simulink model "ANS_GFM_short_term"  (R2021b)
settings: Solver=FixedStepAuto  StartTime=0.0  StopTime=5  FixedStep=Ts  MaxStep=1e-5  RelTol=1e-3
values from neighbouring files (symbols this model uses):
  angle_load = angle(LF.bus(ind_l).Vbus)*180/pi    [init_ANS_GFM_long_term.m]    (also in init_ANS_GFM_short_term.m)
  angleV_LF = Vangle_init/180*pi    [init_ANS_GFM_long_term.m]    (also in init_ANS_GFM_short_term.m)
  awu = 1    [init_ANS_GFM_long_term.m]    (also in init_ANS_GFM_short_term.m)
  C_dc = 1/(Xcdc_pu_or*Zbase_dc_new*100*pi)    [init_ANS_GFM_long_term.m]    (also in init_ANS_GFM_short_term.m)
  C_f = 1/(Xcf_pu_or*Zbase_new*100*pi)    (= 0.013712)    [init_ANS_GFM_long_term.m]    (also in init_ANS_GFM_short_term.m = 0.0141333333333)
  control = 3    [init_ANS_GFM_long_term.m]    (also in init_ANS_GFM_short_term.m = 1)
  D_p = (1/(m_p*w_b))    (= 5209935.26289)    [init_ANS_GFM_long_term.m]    (also in init_ANS_GFM_short_term.m = 5370022.73304)
  Egrid_tmp = 1.054080675694902*400e3    (= 421632.270278)    [init_ANS_GFM_long_term.m]    (also in init_ANS_GFM_short_term.m)
  epsi = 1e-4    (= 0.0001)    [init_ANS_GFM_long_term.m]    (also in init_ANS_GFM_short_term.m)
  eta = m_p*V_m^2    [init_ANS_GFM_long_term.m]    (also in init_ANS_GFM_short_term.m)
  gamma = 2.3    [init_ANS_GFM_long_term.m]    (also in init_ANS_GFM_short_term.m)
  I0_init = [I0_init_a, I0_init_b, I0_init_c]    [init_ANS_GFM_long_term.m]    (also in init_ANS_GFM_short_term.m)
  I_bc = S_bc / (V_bc*sqrt(3))    [init_ANS_GFM_long_term.m]    (also in init_ANS_GFM_short_term.m)
  I_d_int_init = (U_d_int + I_q_int*L_f*w_b - V_d_int - I_d_int*R_f*0)    [init_ANS_GFM_long_term.m]    (also in init_ANS_GFM_short_term.m)
  I_init = [I_init_a, I_init_b, I_init_c]    [init_ANS_GFM_long_term.m]    (also in init_ANS_GFM_short_term.m)
  i_ll = -1.15*(S_bc/Vdc_n)-i_loss_dc    [init_ANS_GFM_long_term.m]    (also in init_ANS_GFM_short_term.m)
  I_max_sat_pu = 1.0 * I_bc *sqrt(2)    [init_ANS_GFM_long_term.m]    (also in init_ANS_GFM_short_term.m)
  I_q_int_init = (U_q_int - I_d_int*L_f*w_b - V_q_int - I_q_int*R_f*0)    [init_ANS_GFM_long_term.m]    (also in init_ANS_GFM_short_term.m)
  i_ul = 1.15*(S_bc/Vdc_n)+i_loss_dc    [init_ANS_GFM_long_term.m]    (also in init_ANS_GFM_short_term.m)
  idppu = 0.95    [init_ANS_GFM_long_term.m]    (also in init_ANS_GFM_short_term.m = 0.92)
  init_dP = -inv(A_pm)*B_pm*dP    [init_ANS_GFM_long_term.m]    (also in init_ANS_GFM_short_term.m)
  init_pm = -inv(A_pm)*B_pm*P_aft    [init_ANS_GFM_long_term.m]    (also in init_ANS_GFM_short_term.m)
  init_tau = -inv(A_tau)*B_tau*idc    [init_ANS_GFM_long_term.m]    (also in init_ANS_GFM_short_term.m)
  J = D_p*tau_f    (= 104198.705258)    [init_ANS_GFM_long_term.m]    (also in init_ANS_GFM_short_term.m = 107400.454661)
  k_dc = eta_1/(Vdc_n*m_p)    [init_ANS_GFM_long_term.m]    (also in init_ANS_GFM_short_term.m)
  K_p = (1/Vdc_n)    [init_ANS_GFM_long_term.m]    (also in init_ANS_GFM_short_term.m)
  K_r = 1/R_dc    [init_ANS_GFM_long_term.m]    (also in init_ANS_GFM_short_term.m)
  Kff_i = 1    [init_ANS_GFM_long_term.m]    (also in init_ANS_GFM_short_term.m)
  Kff_v = 1    [init_ANS_GFM_long_term.m]    (also in init_ANS_GFM_short_term.m)
  Ki_i = (1/n)*1.19    (= 0.0520711785298)    [init_ANS_GFM_long_term.m]    (also in init_ANS_GFM_short_term.m = 0.0505188679245)
  Ki_pll = 4255.3    [init_ANS_GFM_long_term.m]    (also in init_ANS_GFM_short_term.m)
  Ki_v = (n)*1.161022    (= 26.5332227733)    [init_ANS_GFM_long_term.m]    (also in init_ANS_GFM_short_term.m = 27.3485182222)
  ki_v_ac = 2*0.25    (= 0.5)    [init_ANS_GFM_long_term.m]    (also in init_ANS_GFM_short_term.m)
  Kp_i = 0.738891/n    (= 0.032331869895)    [init_ANS_GFM_long_term.m]    (also in init_ANS_GFM_short_term.m = 0.0313680141509)
  Kp_pll = 92    [init_ANS_GFM_long_term.m]    (also in init_ANS_GFM_short_term.m)
  Kp_v = 0.52*n    (= 11.8837333333)    [init_ANS_GFM_long_term.m]    (also in init_ANS_GFM_short_term.m = 12.2488888889)
  kp_v_ac = 0.001    [init_ANS_GFM_long_term.m]    (also in init_ANS_GFM_short_term.m)
  Kpl = 5.0    (= 5)    [init_ANS_GFM_long_term.m]    (also in init_ANS_GFM_short_term.m)
  L1 = cf/sqrt(1+RX^2)*(400e3)^2/Skss/(100*pi)    [init_ANS_GFM_long_term.m]    (also in init_ANS_GFM_short_term.m)
  L_f = Xlf_pu_or*Zbase_new/100/pi    (= 4.37572928821e-06)    [init_ANS_GFM_long_term.m]    (also in init_ANS_GFM_short_term.m = 4.24528301887e-06)
  Lf = 1e6/100/pi    (= 3183.09886184)    [init_ANS_GFM_long_term.m]    (also in init_ANS_GFM_short_term.m = 0.0636619772368)
  m_p = (2*pi*0.5)/(S_bc)    (= 6.10967066042e-10)    [init_ANS_GFM_long_term.m]    (also in init_ANS_GFM_short_term.m = 5.92753330866e-10)
  n = 1/Zb    (= 22.8533333333)    [init_ANS_GFM_long_term.m]    (also in init_ANS_GFM_short_term.m = 23.5555555556)
  P_LF_si = P_LF*S_b    [init_ANS_GFM_long_term.m]    (also in init_ANS_GFM_short_term.m)
  ps = 4440e6/S_bc    (= 0.863477246208)    [init_ANS_GFM_long_term.m]    (also in init_ANS_GFM_short_term.m = 0.837735849057)
  Q_LF_si = Q_LF*S_b    [init_ANS_GFM_long_term.m]    (also in init_ANS_GFM_short_term.m)
  qs = Q_LF*S_b/S_bc    [init_ANS_GFM_long_term.m]    (also in init_ANS_GFM_short_term.m)
  R1 = RX*cf/sqrt(1+RX^2)*(400e3)^2/Skss    [init_ANS_GFM_long_term.m]    (also in init_ANS_GFM_short_term.m)
  R_dc = Rdc_pu_or*Zbase_dc_new    [init_ANS_GFM_long_term.m]    (also in init_ANS_GFM_short_term.m)
  R_f = Rf_pu_or*Zbase_new    (= 2.18786464411e-05)    [init_ANS_GFM_long_term.m]    (also in init_ANS_GFM_short_term.m = 2.12264150943e-05)
  Rf = 1e6    (= 1000000)    [init_ANS_GFM_long_term.m]    (also in init_ANS_GFM_short_term.m = 20)
  S_bc = 5142e6    (= 5142000000)    [init_ANS_GFM_long_term.m]    (also in init_ANS_GFM_short_term.m = 5300000000)
  sat_select = 3    [init_ANS_GFM_long_term.m]    (also in init_ANS_GFM_short_term.m)
  SECM = 3    [init_ANS_GFM_long_term.m]    (also in init_ANS_GFM_short_term.m = 1)
  share_i_load = 1.0    (= 1)    [init_ANS_GFM_long_term.m]    (also in init_ANS_GFM_short_term.m)
  T_en = -0.5    [init_ANS_GFM_long_term.m]    (also in init_ANS_GFM_short_term.m)
  T_off = T_on + 0.1    (= 0.2)    [init_ANS_GFM_long_term.m]    (also in init_ANS_GFM_short_term.m)
  T_on = 0.1    [init_ANS_GFM_long_term.m]    (also in init_ANS_GFM_short_term.m)
  Ts = 2e-6    (= 2e-06)    [init_ANS_GFM_long_term.m]    (also in init_ANS_GFM_short_term.m = 1e-06)
  U_init = [Umag_init_a, Umag_init_b, Umag_init_c]    [init_ANS_GFM_long_term.m]    (also in init_ANS_GFM_short_term.m)
  Uangle_init = angle(V_LF_VSC)*180/pi    [init_ANS_GFM_long_term.m]    (also in init_ANS_GFM_short_term.m)
  Umag_init = abs(V_LF_VSC)*V_bc*sqrt(2/3)    [init_ANS_GFM_long_term.m]    (also in init_ANS_GFM_short_term.m)
  V1_rms = 15e3    (= 15000)    [init_ANS_GFM_long_term.m]    (also in init_ANS_GFM_short_term.m)
  V_d_int = abs(V_LF)*V_bc*sqrt(2/3)    [init_ANS_GFM_long_term.m]    (also in init_ANS_GFM_short_term.m)
  V_d_int_init = (I_d_int + V_q_int*C_f*w_b - I0_d_int)    [init_ANS_GFM_long_term.m]    (also in init_ANS_GFM_short_term.m)
  V_init = [V_init_a, V_init_b, V_init_c]    [init_ANS_GFM_long_term.m]    (also in init_ANS_GFM_short_term.m)
  V_m = sqrt(2/3)*V_bc    [init_ANS_GFM_long_term.m]    (also in init_ANS_GFM_short_term.m)
  V_q_int_init = (I_q_int - V_d_int*C_f*w_b - I0_q_int)    [init_ANS_GFM_long_term.m]    (also in init_ANS_GFM_short_term.m)
  Vdc_n = 3*V_m    [init_ANS_GFM_long_term.m]    (also in init_ANS_GFM_short_term.m)
  Vref = V_LF_mag*V_m    [init_ANS_GFM_long_term.m]    (also in init_ANS_GFM_short_term.m)
  w_b = 2*pi*f_b    (= 314.159265359)    [init_ANS_GFM_long_term.m]    (also in init_ANS_GFM_short_term.m)
  w_f = 2*pi*5    (= 31.4159265359)    [init_ANS_GFM_long_term.m]    (also in init_ANS_GFM_short_term.m)
  Zbase_new = V1_rms^2/S_bc    (= 0.0437572928821)    [init_ANS_GFM_long_term.m]    (also in init_ANS_GFM_short_term.m = 0.0424528301887)
undefined symbols (not defined in the file or in its folder): A_pm, A_tau, B_pm, B_tau, C_pm, C_tau, D_pm, D_tau, find_system, idq0_init, Pm, sm_init, v_d, v_q, Ve
libraries: spsBreakerLib x270, spsGroundLib x21, spsThreePhaseSeriesRLCBranchLib x12, spsabctodq0Lib x11, simulink x9, spsEdgeDetectorLib x8, spsThreePhaseVIMeasurementLib x7, spsLoadFlowBusLib x7, spsSeriesRLCBranchLib x6, spsControlledVoltageSourceLib x6, spsCurrentMeasurementLib x6, spsVoltageMeasurementLib x6
(part 6 of 7)

== system ANS_GFM_short_term/OLTC for load flow/OLTCC1 ==
  note: R2
  note: R1
  note: Transfer Switch
  Demux : Demux  Outputs=21
      settings: DisplayOption=none
  Display : Display
  Display1 : Display
  "Sw0 " : spsBreakerLib/Breaker  InitialState=InitialStates(1)  SwitchingTimes="[ 1/60  5/60 ]"  External=on  BreakerResistance=1e-6  SnubberResistance=1e8  SnubberCapacitance=inf  Measurements=None  MoreParameters=off  NoBreakLoop=off
      settings: SourceProductBaseCode=PS
  "Sw1 " : spsBreakerLib/Breaker  InitialState=InitialStates(2)  SwitchingTimes="[ 1/60  5/60 ]"  External=on  BreakerResistance=1e-4  SnubberResistance=1e6  SnubberCapacitance=inf  Measurements=None  MoreParameters=off  NoBreakLoop=off
      settings: SourceProductBaseCode=PS
  Sw10 : spsBreakerLib/Breaker  InitialState=InitialStates(11)  SwitchingTimes="[ 1/60  5/60 ]"  External=on  BreakerResistance=1e-6  SnubberResistance=1e8  SnubberCapacitance=inf  Measurements=None  MoreParameters=off  NoBreakLoop=off
      settings: SourceProductBaseCode=PS
  Sw11 : spsBreakerLib/Breaker  InitialState=InitialStates(12)  SwitchingTimes="[ 1/60  5/60 ]"  External=on  BreakerResistance=1e-6  SnubberResistance=1e8  SnubberCapacitance=inf  Measurements=None  MoreParameters=off  NoBreakLoop=off
      settings: SourceProductBaseCode=PS
  Sw12 : spsBreakerLib/Breaker  InitialState=InitialStates(13)  SwitchingTimes="[ 1/60  5/60 ]"  External=on  BreakerResistance=1e-6  SnubberResistance=1e8  SnubberCapacitance=inf  Measurements=None  MoreParameters=off  NoBreakLoop=off
      settings: SourceProductBaseCode=PS
  Sw13 : spsBreakerLib/Breaker  InitialState=InitialStates(14)  SwitchingTimes="[ 1/60  5/60 ]"  External=on  BreakerResistance=1e-4  SnubberResistance=1e6  SnubberCapacitance=inf  Measurements=None  MoreParameters=off  NoBreakLoop=off
      settings: SourceProductBaseCode=PS
  Sw14 : spsBreakerLib/Breaker  InitialState=InitialStates(15)  SwitchingTimes="[ 1/60  5/60 ]"  External=on  BreakerResistance=1e-4  SnubberResistance=1e6  SnubberCapacitance=inf  Measurements=None  MoreParameters=off  NoBreakLoop=off
      settings: SourceProductBaseCode=PS
  Sw15 : spsBreakerLib/Breaker  InitialState=InitialStates(16)  SwitchingTimes="[ 1/60  5/60 ]"  External=on  BreakerResistance=1e-4  SnubberResistance=1e6  SnubberCapacitance=inf  Measurements=None  MoreParameters=off  NoBreakLoop=off
      settings: SourceProductBaseCode=PS
  Sw16 : spsBreakerLib/Breaker  InitialState=InitialStates(17)  SwitchingTimes="[ 1/60  5/60 ]"  External=on  BreakerResistance=1e-4  SnubberResistance=1e6  SnubberCapacitance=inf  Measurements=None  MoreParameters=off  NoBreakLoop=off
      settings: SourceProductBaseCode=PS
  Sw17 : spsBreakerLib/Breaker  InitialState=InitialStates(18)  SwitchingTimes="[ 1/60  5/60 ]"  External=on  BreakerResistance=1e-4  SnubberResistance=1e6  SnubberCapacitance=inf  Measurements=None  MoreParameters=off  NoBreakLoop=off
      settings: SourceProductBaseCode=PS
  Sw18 : spsBreakerLib/Breaker  InitialState=InitialStates(19)  SwitchingTimes="[ 1/60  5/60 ]"  External=on  BreakerResistance=1e-4  SnubberResistance=1e6  SnubberCapacitance=inf  Measurements=None  MoreParameters=off  NoBreakLoop=off
      settings: SourceProductBaseCode=PS
  Sw19 : spsBreakerLib/Breaker  InitialState=InitialStates(20)  SwitchingTimes="[ 1/60  5/60 ]"  External=on  BreakerResistance=1e-4  SnubberResistance=1e6  SnubberCapacitance=inf  Measurements=None  MoreParameters=off  NoBreakLoop=off
      settings: SourceProductBaseCode=PS
  "Sw2 " : spsBreakerLib/Breaker  InitialState=InitialStates(3)  SwitchingTimes="[ 1/60  5/60 ]"  External=on  BreakerResistance=1e-4  SnubberResistance=1e6  SnubberCapacitance=inf  Measurements=None  MoreParameters=off  NoBreakLoop=off
      settings: SourceProductBaseCode=PS
  Sw20 : spsBreakerLib/Breaker  InitialState=InitialStates(21)  SwitchingTimes="[ 1/60  5/60 ]"  External=on  BreakerResistance=1e-4  SnubberResistance=1e6  SnubberCapacitance=inf  Measurements=None  MoreParameters=off  NoBreakLoop=off
      settings: SourceProductBaseCode=PS
  "Sw3 " : spsBreakerLib/Breaker  InitialState=InitialStates(4)  SwitchingTimes="[ 1/60  5/60 ]"  External=on  BreakerResistance=1e-4  SnubberResistance=1e6  SnubberCapacitance=inf  Measurements=None  MoreParameters=off  NoBreakLoop=off
      settings: SourceProductBaseCode=PS
  "Sw4 " : spsBreakerLib/Breaker  InitialState=InitialStates(5)  SwitchingTimes="[ 1/60  5/60 ]"  External=on  BreakerResistance=1e-4  SnubberResistance=1e6  SnubberCapacitance=inf  Measurements=None  MoreParameters=off  NoBreakLoop=off
      settings: SourceProductBaseCode=PS
  "Sw5 " : spsBreakerLib/Breaker  InitialState=InitialStates(6)  SwitchingTimes="[ 1/60  5/60 ]"  External=on  BreakerResistance=1e-4  SnubberResistance=1e6  SnubberCapacitance=inf  Measurements=None  MoreParameters=off  NoBreakLoop=off
      settings: SourceProductBaseCode=PS
  "Sw6 " : spsBreakerLib/Breaker  InitialState=InitialStates(7)  SwitchingTimes="[ 1/60  5/60 ]"  External=on  BreakerResistance=1e-6  SnubberResistance=1e8  SnubberCapacitance=inf  Measurements=None  MoreParameters=off  NoBreakLoop=off
      settings: SourceProductBaseCode=PS
  "Sw7 " : spsBreakerLib/Breaker  InitialState=InitialStates(8)  SwitchingTimes="[ 1/60  5/60 ]"  External=on  BreakerResistance=1e-6  SnubberResistance=1e68  SnubberCapacitance=inf  Measurements=None  MoreParameters=off  NoBreakLoop=off
      settings: SourceProductBaseCode=PS
  "Sw8 " : spsBreakerLib/Breaker  InitialState=InitialStates(9)  SwitchingTimes="[ 1/60  5/60 ]"  External=on  BreakerResistance=1e-6  SnubberResistance=1e8  SnubberCapacitance=inf  Measurements=None  MoreParameters=off  NoBreakLoop=off
      settings: SourceProductBaseCode=PS
  Sw9 : spsBreakerLib/Breaker  InitialState=InitialStates(10)  SwitchingTimes="[ 1/60  5/60 ]"  External=on  BreakerResistance=1e-6  SnubberResistance=1e8  SnubberCapacitance=inf  Measurements=None  MoreParameters=off  NoBreakLoop=off
      settings: SourceProductBaseCode=PS
  SwR1 : spsBreakerLib/Breaker  InitialState=1  SwitchingTimes="[ 1/60  5/60 ]"  External=on  BreakerResistance=1e-6  SnubberResistance=Rtransfer  SnubberCapacitance=inf  Measurements=None  MoreParameters=off  NoBreakLoop=off
      settings: SourceProductBaseCode=PS
  SwR2 : spsBreakerLib/Breaker  InitialState=1  SwitchingTimes="[ 1/60  5/60 ]"  External=on  BreakerResistance=1e-6  SnubberResistance=Rtransfer  SnubberCapacitance=inf  Measurements=None  MoreParameters=off  NoBreakLoop=off
      settings: SourceProductBaseCode=PS
  Tapped Winding Inversion : Subsystem
  Tap20 : PMIOPort  Side=Right
  Tap19 : PMIOPort  Port=2  Side=Right
  Tap18 : PMIOPort  Port=3  Side=Right
  Tap17 : PMIOPort  Port=4  Side=Right
  Tap16 : PMIOPort  Port=5  Side=Right
  Tap15 : PMIOPort  Port=6  Side=Right
  Tap14 : PMIOPort  Port=7  Side=Right
  Tap13 : PMIOPort  Port=8  Side=Right
  Tap12 : PMIOPort  Port=9  Side=Right
  Tap11 : PMIOPort  Port=10  Side=Right
  Tap10 : PMIOPort  Port=11  Side=Right
  Tap9 : PMIOPort  Port=12  Side=Right
  Tap8 : PMIOPort  Port=13  Side=Right
  Tap7 : PMIOPort  Port=14  Side=Right
  Tap6 : PMIOPort  Port=15  Side=Right
  Tap5 : PMIOPort  Port=16  Side=Right
  Tap4 : PMIOPort  Port=17  Side=Right
  Tap3 : PMIOPort  Port=18  Side=Right
  Tap2 : PMIOPort  Port=19  Side=Right
  Tap1 : PMIOPort  Port=20  Side=Right
  Tap0 : PMIOPort  Port=21  Side=Right
  W2+ : PMIOPort  Port=22  Side=Right
  Out : PMIOPort  Port=23  Side=Left
  wires:
  Demux/9 -> "Sw8 "/1
  Demux/8 -> "Sw7 "/1
  Demux/7 -> Display/1, "Sw6 "/1
  Demux/6 -> "Sw5 "/1
  Demux/5 -> "Sw4 "/1
  Demux/4 -> "Sw3 "/1
  Demux/3 -> "Sw2 "/1
  Demux/2 -> "Sw1 "/1
  Demux/1 -> "Sw0 "/1
  [SwInversion] -> Tapped Winding Inversion/1(Inv)
  [SwTransfer] -> SwR2/1, SwR1/1
  [SwSelect] -> Demux/1, Display1/1
  Demux/10 -> Sw9/1
  Demux/11 -> Sw10/1
  Demux/12 -> Sw11/1
  Demux/13 -> Sw12/1
  Demux/14 -> Sw13/1
  Demux/15 -> Sw14/1
  Demux/16 -> Sw15/1
  Demux/17 -> Sw16/1
  Demux/18 -> Sw17/1
  Demux/19 -> Sw18/1
  Demux/20 -> Sw19/1
  Demux/21 -> Sw20/1
  connections:
  "Sw0 "/LConn1 -- Tap0/RConn1 -- Tapped Winding Inversion/LConn2
  Tap1/RConn1 -- "Sw1 "/LConn1
  Tap2/RConn1 -- "Sw2 "/LConn1
  Tap6/RConn1 -- "Sw6 "/LConn1
  Tap4/RConn1 -- "Sw4 "/LConn1
  Tap5/RConn1 -- "Sw5 "/LConn1
  SwR1/RConn1 -- Tapped Winding Inversion/LConn1 -- SwR2/RConn1
  SwR2/LConn1 -- Sw19/RConn1 -- Sw17/RConn1 -- Sw15/RConn1 -- Sw13/RConn1 -- Sw11/RConn1 -- Sw9/RConn1 -- "Sw7 "/RConn1 -- "Sw5 "/RConn1 -- "Sw3 "/RConn1 -- "Sw1 "/RConn1
  Tapped Winding Inversion/RConn1 -- Out/RConn1
  W2+/RConn1 -- Tapped Winding Inversion/RConn2
  "Sw6 "/RConn1 -- "Sw4 "/RConn1 -- "Sw2 "/RConn1 -- "Sw0 "/RConn1 -- Sw20/RConn1 -- Sw18/RConn1 -- Sw16/RConn1 -- Sw14/RConn1 -- Sw12/RConn1 -- Sw10/RConn1 -- "Sw8 "/RConn1 -- SwR1/LConn1
  Tap3/RConn1 -- "Sw3 "/LConn1
  Tap8/RConn1 -- "Sw8 "/LConn1
  Tap7/RConn1 -- "Sw7 "/LConn1
  Tap9/RConn1 -- Sw9/LConn1
  Tap10/RConn1 -- Sw10/LConn1
  Tap11/RConn1 -- Sw11/LConn1
  Tap13/RConn1 -- Sw13/LConn1
  Tap12/RConn1 -- Sw12/LConn1
  Tap14/RConn1 -- Sw14/LConn1
  Tap15/RConn1 -- Sw15/LConn1
  Tap16/RConn1 -- Sw16/LConn1
  Tap17/RConn1 -- Sw17/LConn1
  Tap18/RConn1 -- Sw18/LConn1
  Tap19/RConn1 -- Sw19/LConn1
  Tap20/RConn1 -- Sw20/LConn1

== system ANS_GFM_short_term/OLTC for load flow/Subsystem ==
  note: A) Open the Three-Phase OLTC Transformer  mask (use Edit/Edit mask)
      |      In Initialization section, modify 1st line as below:
      |                   NumberOfTaps=10;
      |
      | B) Open the TransformerA block dialog box inside the Three-Phase OLTC Transformer (use Edit/Look under mask)
      |      and change the 'Number of Taps' parameter  from 7 to 9 (adding two intermediate taps on upper left winding (winding 1)).
      |
      | C) Open the  OLTCA block inside the Three-Phase OLTC Transformer (use Edit/Look under mask) and make the following changes:
      |       1) Open the dialog box of the Demux block and change the parameter  'Number of outputs' from 9 to 11.
      |       2) Add 2 switches labeled Sw9 and Sw10 (duplicate Sw8 block); Position these two blocks on top of Sw8 block.
      |       3) Open the dialog box of Sw9 and Sw10 blocks and change the  parameter "Initial state" as follows:
      |              Sw9 --> InitialState(10)
      |              Sw10-->InitialState(11)
      |      4) Add two connection ports labeled  respectively Tap9 and Tap10 (duplicate Tap8 block). Position these two blocks on top of Tap8 block.
      |      5) Renumber ALL connection ports as follows:
      |         Open dialog box of each connection port and change  'Port number' and  'Port location' parameters as in the table below.
      |         (all port locations should be set to  'right' except for 'Out' port which must be 'left')
      |         Start the renumbering with the top port  labeled Tap10.
      |
      |            Port           Port          Port
      |            label       number   location
      |           ---------    -----------    -----------
      |            Tap10       1               right
      |            Tap9         2               right
      |            .....            ......              .......
      |            Tap 1       11               right
      |            Tap 0       12               right
      |            W2+         13               right
      |            Out           14               left
      |
      |     6) Connect terminal 1 of Sw9 and Sw10 respectively to ports labeled Tap10 (port #1)  and Tap9  (port #2)
      |     7) Connect terminal 2 of Sw9 and Sw10 respectively to nodes labeled R2 and R1
      |     8) Close the OLTCA block.
      |
      | D)  Connect the Tap10, Tap9 ...Tap0 connectors of OLTCA respectively to  1+, 1.1,   ... 1 connectors of tapped winding of TransformerA.
      |
      | E)  Cut  the OLTCB and OLTCC blocks and replace them with a duplicate of OLTCA block.  Rename these two blocks OLTCB and OLTCC.
      |
      | F)  Cut  the TransformerB and TransformerC blocks and replace them with a duplicate of TransformerA block. Rename these two blocks TransformerB and TransformerC.
      |
      | G) Make connections between OLTC to Transformer for  phases B and C as for phase A.
      |
      | H) Ckeck that the secondary windings of  the three transformers are connected in Delta (D1)
  note: The following procedure explains how to increase the number of taps from 8 (17 OLTC positions)  to 10  (21 OLTC positions)
      |    If you want to decrease the number of taps, follow the reverse procedure (Change 'add' to ' cut'  and skip step C3).

== system ANS_GFM_short_term/OLTC for load flow/Voltage regulator ==
  Vmes (pu) : Inport
  Ready : Inport  Port=2
  RegOn : Inport  Port=3
  Dead Zone : DeadZone  LowerValue=-DeadBand/2  UpperValue=+DeadBand/2  SaturateOnIntegerOverflow=on
  Logical Operator : Logic  AllPortsSameDT=off
  Logical Operator1 : Logic  AllPortsSameDT=off
  MyDelay1 : Subsystem
  MyDelay2 : Subsystem
  Relational Operator : RelationalOperator  Operator=>  RndMeth=Nearest
  Relational Operator1 : RelationalOperator  Operator=<  RndMeth=Nearest
  Sum : Sum  Inputs=|+-  SaturateOnIntegerOverflow=on
  Switch : Switch  Threshold=1.5  SaturateOnIntegerOverflow=on
  Transport Delay : TransportDelay  DelayTime=Ts  InitialOutput=1
  Vref : Constant  Value=Vref
  Vref1 : Constant  Value=0
  Vref2 : Constant  Value=0
  Vref3 : Constant  Value=0
  Up : Outport  VectorParamsAs1DForOutWhenUnconnected=off
  Down : Outport  Port=2  VectorParamsAs1DForOutWhenUnconnected=off
  wires:
  Vref2/1 -> Switch/3
  RegOn/1 -> Switch/2
  Switch/1 -> Dead Zone/1
  Sum/1 -> Switch/1
  Vref/1 -> Sum/1
  Vmes (pu)/1 -> Sum/2
  Dead Zone/1 -> Relational Operator1/1, Relational Operator/1
  Vref1/1 -> Relational Operator/2
  Relational Operator/1 -> Logical Operator/1
  Ready/1 -> Transport Delay/1
  Transport Delay/1 -> Logical Operator1/1, Logical Operator/2
  Relational Operator1/1 -> Logical Operator1/2
  Logical Operator1/1 -> MyDelay1/1(in)
  Vref3/1 -> Relational Operator1/2
  MyDelay2/1(out) -> Up/1
  MyDelay1/1(out) -> Down/1
  Logical Operator/1 -> MyDelay2/1(in)

== system ANS_GFM_short_term/Synchronous Generator(GENTPJ)/AVR+OEL+PSS ==
  ie : Inport
  ut : Inport  Port=2
  xspeed : Inport  Port=3
  Array logic : Subsystem
  Constant : Constant  Value=ifdlim
  Constant2 : Constant  Value=uref+ve0/G
  Constant3 : Constant  Value=PSS_act
  Constant4 : Constant  Value=0
  DT1-Glied : Subsystem  mask(State Space Model){A=-2/30, B=1, C=-1/3, D=5, x_init=-1*1/(-2/30)}
      mask prompts: x_init "Initialisierung (x_init)"
      mask help:
      | [A,B,C,D] = tf2ss([Kp],[Tw 1])
      |
      | Kp = 75
      | Tw = 15
      |
      | Initialisierung:
      |
      | x_init = -B*u/A
      |
      | --> u muss man zurückverfolgen, welchen Wert dieser hat
  Gain : Gain  Gain=-1
  Gain2 : Gain  Gain=10
  Integrator Limited : Integrator  InitialCondition=L1  LimitOutput=on  LowerSaturationLimit=L1
  Integrator Limited1 : Integrator  InitialCondition=ve0  LimitOutput=on  UpperSaturationLimit=L2  LowerSaturationLimit=0
  Lead-Lag : Subsystem  mask(State Space Model){A=-0.08, B=1, C=5.76, D=48, x_init=-1*ve0/G/(-0.08)}
      mask prompts: x_init "Initialisierung (x_init)"
      mask help:
      | [A,B,C,D] = tf2ss(120*[5 1],[12.5 1])
      |
      | Initialisierung:
      |
      | x_init = -B*u/A
      |
      | --> u muss man zurückverfolgen, welchen Wert dieser hat
  Lead_Lag1 : Subsystem  mask(State Space Model){A=-83-1/3, B=1, C=-1.4444e+03, D=18+1/3, x_init=-1*0/(-83-1/3)}
      mask prompts: x_init "Initialisierung (x_init)"
      mask help:
      | [A,B,C,D] = tf2ss([T1 1],[T2 1])
      |
      | T1 = 0.22
      | T2 = 0.012
      |
      | Initialisierung:
      |
      | x_init = -B*u/A
      |
      | --> u muss man zurückverfolgen, welchen Wert dieser hat
  Lead_Lag2 : Subsystem  mask(State Space Model){A=-83-1/3, B=1, C=-1.4444e+03, D=18+1/3, x_init=-1*0/(-83-1/3)}
      mask prompts: x_init "Initialisierung (x_init)"
      mask help:
      | [A,B,C,D] = tf2ss([T1 1],[T2 1])
      |
      | T1 = 0.22
      | T2 = 0.012
      |
      | Initialisierung:
      |
      | x_init = -B*u/A
      |
      | --> u muss man zurückverfolgen, welchen Wert dieser hat
  Min : MinMax  Inputs=2
  Mux : Mux  Commented=on  Inputs=2
  Saturation : Saturate  UpperLimit=C  LowerLimit=-C
  Sum : Sum  Inputs=|+-
  Sum1 : Sum  Inputs=+-+
  Sum2 : Sum  Inputs=|+-
  Switch1 : Switch  Criteria=u2 > Threshold
  Switch2 : Switch  Criteria=u2 > Threshold
  To Workspace : ToWorkspace  Commented=on  VariableName=oel  SaveFormat=Timeseries  SampleTime=-1
      settings: Decimation=100
  Transfer Fcn : TransferFcn  Commented=on  Numerator=[Ta 1]  Denominator=[Tb 1]
  Transfer Fcn1 : TransferFcn  Commented=on  Numerator=[Kp]  Denominator=[Tw 1]
  Transfer Fcn2 : TransferFcn  Commented=on  Numerator=[T1 1]  Denominator=[T2 1]
  Transfer Fcn3 : TransferFcn  Commented=on  Numerator=[T1 1]  Denominator=[T2 1]
  ve : Outport
  wires:
  Sum/1 -> Array logic/1(u), Gain/1
  Gain2/1 -> Integrator Limited1/1
  Sum1/1 -> Switch1/3, Min/2
  Integrator Limited1/1 -> ve/1, Sum2/2
  Switch2/1 -> Sum1/3
  Array logic/1(y) -> Mux/1, Integrator Limited/1
  Constant3/1 -> Switch2/2
  Saturation/1 -> Switch2/1
  Constant4/1 -> Switch2/3
  Min/1 -> Lead-Lag/1(u)
  Constant/1 -> Sum/2
  Integrator Limited/1 -> Mux/2, Switch1/2
  Gain/1 -> Switch1/1
  Switch1/1 -> Min/1
  ie/1 -> Sum/1
  Sum2/1 -> Gain2/1
  ut/1 -> Sum1/2
  Constant2/1 -> Sum1/1
  Lead-Lag/1(y) -> Sum2/1
  Transfer Fcn1/1 -> Transfer Fcn2/1
  Transfer Fcn2/1 -> Transfer Fcn3/1
  xspeed/1 -> DT1-Glied/1(u)
  DT1-Glied/1(y) -> Lead_Lag1/1(u)
  Lead_Lag1/1(y) -> Lead_Lag2/1(u)
  Lead_Lag2/1(y) -> Saturation/1
  Mux/1 -> To Workspace/1

== system ANS_GFM_short_term/Synchronous Generator(GENTPJ)/Grid Interface ==
  Vdterm : Inport
  Vqterm : Inport  Port=2
  wt : Inport  Port=3
  Constant : Constant  Value=0
  Delay : Delay  DelayLength=1  InitialCondition=idq0_init
  Delay1 : Delay  DelayLength=1  InitialCondition=[v_d v_q 0]
  Demux{1..4} (4 alike) : Demux  Outputs=3
  Dot Product : DotProduct  InputSameDT=on  OutDataTypeStr=Inherit: Inherit via internal rule
  GENTPJ_U1 : spsControlledVoltageSourceLib/Controlled Voltage Source  Initialize=on  Source_Type=AC  Amplitude=Urmsinit*sqrt(2)/sqrt(3)  Phase=phiinit  Frequency=50  Measurements=None
  GENTPJ_U2 : spsControlledVoltageSourceLib/Controlled Voltage Source  Initialize=on  Source_Type=AC  Amplitude=Urmsinit*sqrt(2)/sqrt(3)  Phase=phiinit-120  Frequency=50  Measurements=None
  GENTPJ_U3 : spsControlledVoltageSourceLib/Controlled Voltage Source  Initialize=on  Source_Type=AC  Amplitude=Urmsinit*sqrt(2)/sqrt(3)  Phase=phiinit+120  Frequency=50  Measurements=None
  Gain : Gain  Gain=Sbase_grid/Sbase
  Gain1 : Gain  Gain=Urms*sqrt(2/3)
  Gain2 : Gain  Gain=sqrt(2)
  Gain3 : Gain  Gain=Ra
  Gain4 : Gain  Gain=Xl
  Gain5 : Gain  Gain=Ra
  Gain6 : Gain  Gain=Xl
  Ground1 : spsGroundLib/Ground  LConnTagsString=a
  LF_GENTPJ : spsThreePhaseProgrammableVoltageSourceLib/Three-Phase Programmable Voltage Source  Commented=on  PositiveSequence=[(15000)*1 -11.7888 50]  VariationEntity=None  VariationType=Table of time-amplitude pairs  VariationTypeAlt=Step  VariationStep=0.2  VariationRate=10  VariationMagnitude=0.3  VariationFrequency=2  VariationTiming="[5  20]"  VariationPhaseA=off  Amplitudes=[ 1 ]  TimeValues=[0]  HarmonicGeneration=off  HarmonicA=[3 0.2 -25 0]  HarmonicB=[2 0.15 35 2]  Timing="[0.05  3]"  BusType=PV  Pref=4400000000  Qref=0  Qmin=-2956145970.6855  Qmax=2956145970.6855
  Load Flow Bus : spsLoadFlowBusLib/Load Flow Bus  LConnTagsString=a  Phases=single  Connectors=on one side  ID=GENTPJ  Vbase=Urms  Vref=1  Vangle=0  VLF=1  VLFb=1  VLFc=1  angleLF=-11.79  angleLFb=0  angleLFc=0
      settings: SourceProductBaseCode=PS
  Mux1 : Mux  Inputs=3
  RMS3 : spsRMSLib/RMS  TrueRMS=off  Freq=50  RMSInit=1/sqrt(2)  Ts=0
  Sqrt : Sqrt  SaturateOnIntegerOverflow=on
  Sqrt1 : Sqrt  SaturateOnIntegerOverflow=on
  Square : Math  Operator=square  SaturateOnIntegerOverflow=on
  Square1 : Math  Operator=square  SaturateOnIntegerOverflow=on
  Sum : Sum  Inputs=++-
  Sum1 : Sum  Inputs=+++
  Sum2 : Sum  Inputs=|++
  Terminator{,1..3} (4 alike) : Terminator
  Three-Phase V-I Measurement : spsThreePhaseVIMeasurementLib/Three-Phase V-I Measurement  VoltageMeasurement=phase-to-ground  SetLabelV=off  LabelV=Vabc  Vpu=on  VpuLL=off  CurrentMeasurement=yes  SetLabelI=off  LabelI=Iabc  Ipu=on  Pbase=Sbase_grid  Vbase=Urms  OutputType=Complex  PhasorSimulation=off  PSBequivalent=0
  abc to dq0 : spsabctodq0Lib/abc to dq0  Alignment=90 degrees behind phase A axis
  abc to dq1 : spsabctodq0Lib/abc to dq0  Alignment=90 degrees behind phase A axis
  dq0 to abc : spsdq0toabcLib/dq0 to abc  Alignment=90 degrees behind phase A axis
  a : PMIOPort  Side=Right
  b : PMIOPort  Port=2  Side=Right
  c : PMIOPort  Port=3  Side=Right
  id : Outport
  iq : Outport  Port=2
  El : Outport  Port=3
  |Uterm| : Outport  Port=4
  tag scope: V_SM=global
  wires:
  Three-Phase V-I Measurement/2 -> abc to dq0/1
  Demux1/1 -> GENTPJ_U1/1
  Demux1/3 -> GENTPJ_U3/1
  Vqterm/1 -> Mux1/2
  wt/1 -> dq0 to abc/2, abc to dq1/2, abc to dq0/2
  Demux1/2 -> GENTPJ_U2/1
  dq0 to abc/1 -> Demux1/1
  Constant/1 -> Mux1/3
  Vdterm/1 -> Mux1/1
  Demux2/3 -> Terminator/1
  abc to dq0/1 -> Gain/1
  Demux2/1 -> Gain6/1, id/1, Gain3/1
  Delay/1 -> Demux2/1
  Gain/1 -> Delay/1
  Mux1/1 -> Gain1/1
  Gain1/1 -> dq0 to abc/1
  Three-Phase V-I Measurement/1 -> Demux4/1, abc to dq1/1
  Demux3/1 -> Sum/2
  Gain3/1 -> Sum/1
  Gain4/1 -> Sum/3
  Sum/1 -> Square/1
  Demux3/2 -> Sum1/2
  Gain5/1 -> Sum1/1
  Demux2/2 -> Gain5/1, iq/1, Gain4/1
  Gain6/1 -> Sum1/3
  Sum1/1 -> Square1/1
  Square/1 -> Sum2/1
  Square1/1 -> Sum2/2
  Demux3/3 -> Terminator1/1
  Sum2/1 -> Sqrt1/1
  Delay1/1 -> Dot Product/2, Dot Product/1, Demux3/1
  Sqrt1/1 -> El/1
  abc to dq1/1 -> Delay1/1
  Dot Product/1 -> Sqrt/1
  Sqrt/1 -> |Uterm|/1
  Gain2/1 -> [V_SM]
  RMS3/1 -> Gain2/1
  Demux4/1 -> RMS3/1
  Demux4/2 -> Terminator2/1
  Demux4/3 -> Terminator3/1
  connections:
  Ground1/LConn1 -- LF_GENTPJ/LConn1 -- GENTPJ_U3/LConn1 -- GENTPJ_U1/LConn1 -- GENTPJ_U2/LConn1
  GENTPJ_U1/RConn1 -- LF_GENTPJ/RConn1 -- Load Flow Bus/LConn1 -- Three-Phase V-I Measurement/LConn1
  GENTPJ_U2/RConn1 -- LF_GENTPJ/RConn2 -- Three-Phase V-I Measurement/LConn2
  Three-Phase V-I Measurement/RConn3 -- c/RConn1
  GENTPJ_U3/RConn1 -- LF_GENTPJ/RConn3 -- Three-Phase V-I Measurement/LConn3
  Three-Phase V-I Measurement/RConn1 -- a/RConn1
  Three-Phase V-I Measurement/RConn2 -- b/RConn1

== system ANS_GFM_short_term/Synchronous Generator(GENTPJ)/Mechanical Equations ==
  Pm : Inport
  Te : Inport  Port=2
  Divide : Product  Inputs=/*
  Gain1 : Gain  Gain=D
  Gain2 : Gain  Gain=1/(2*H)
  Gain3 : Gain  Gain=100*pi
  Gain4 : Gain  Gain=100*pi
  Gain5 : Gain  Gain=180/pi
  Integrator : Integrator
  Integrator1 : Integrator  InitialCondition=delta0_init
  Integrator2 : Integrator  InitialCondition=delta0_init*180/pi
  Sum : Sum  Inputs=+-
  Sum1 : Sum  Inputs=-+|
  Sum2 : Sum  Inputs=++|
  nominal speed : Constant
  1+w : Outport
  wt : Outport  Port=2
  delta : Outport  Port=3
  wires:
  Integrator1/1 -> wt/1
  Te/1 -> Sum/2
  Integrator/1 -> Gain3/1, Sum2/2, Gain1/1
  Gain4/1 -> Integrator1/1
  Gain2/1 -> Integrator/1
  Sum2/1 -> 1+w/1, Divide/1, Gain4/1
  Gain3/1 -> Gain5/1
  Sum1/1 -> Divide/2
  nominal speed/1 -> Sum2/1
  Gain1/1 -> Sum1/1
  Sum/1 -> Gain2/1
  Pm/1 -> Sum1/2
  Divide/1 -> Sum/1
  Integrator2/1 -> delta/1
  Gain5/1 -> Integrator2/1

== system ANS_GFM_short_term/Synchronous Generator(GENTPJ)/Power calculation ==
  1+w : Inport
  Vdterm : Inport  Port=2
  Vqterm : Inport  Port=3
  Id : Inport  Port=4
  Iq : Inport  Port=5
  Divide : Product  Inputs=*/
  Gain1 : Gain  Gain=Ra
  Gain2 : Gain  Gain=Ra
  Product : Product
  Product1 : Product
  Sum : Sum  Inputs=|++
  Sum1 : Sum  Inputs=|++
  Sum2 : Sum  Inputs=|++
  Te : Outport
  wires:
  Gain1/1 -> Sum/2
  Sum1/1 -> Product1/1
  Sum2/1 -> Divide/1
  Gain2/1 -> Sum1/2
  Product/1 -> Sum2/1
  Vdterm/1 -> Sum/1
  Product1/1 -> Sum2/2
  Id/1 -> Product/2, Gain1/1
  Iq/1 -> Product1/2, Gain2/1
  Divide/1 -> Te/1
  Sum/1 -> Product/1
  Vqterm/1 -> Sum1/1
  1+w/1 -> Divide/2

== system ANS_GFM_short_term/Synchronous Generator(GENTPJ)/Rotor Equations ==
  ve : Inport
  id : Inport  Port=2
  iq : Inport  Port=3
  El : Inport  Port=4
  1+Sd : Subsystem
  1+Sd1 : Subsystem
  1+Sq1 : Subsystem
  1+Sq2 : Subsystem
  Gain1 : Gain  Gain=1/Td0s
  Gain10 : Gain  Gain=(Xqs-Xqss)
  Gain2 : Gain  Gain=(Xd-Xdss)/(Xds-Xdss)
  Gain3 : Gain  Gain=(Xd-Xds)/(Xds-Xdss)
  Gain4 : Gain  Gain=1/Td0ss
  Gain5 : Gain  Gain=(Xds-Xdss)
  Gain6 : Gain  Gain=1/Tq0s
  Gain7 : Gain  Gain=(Xq-Xqss)/(Xqs-Xqss)
  Gain8 : Gain  Gain=(Xq-Xqs)/(Xqs-Xqss)
  Gain9 : Gain  Gain=1/Tq0ss
  Integrator : Integrator  InitialCondition=eqs
  Integrator1 : Integrator  InitialCondition=eqss
  Integrator2 : Integrator  InitialCondition=eds
  Integrator3 : Integrator  InitialCondition=edss
  Sum : Sum  Inputs=++-
  Sum1 : Sum  Inputs=-+
  Sum2 : Sum  Inputs=-+-
  Sum3 : Sum  Inputs=+-
  Sum5 : Sum  Inputs=-++
  ifd : Outport
  Edss : Outport  Port=2
  Eqss : Outport  Port=3
  wires:
  1+Sd/1(y) -> Gain2/1, Sum2/2
  Gain1/1 -> Integrator/1
  Gain3/1 -> Sum/1, Sum1/1
  Gain2/1 -> Sum/3, Sum1/2
  1+Sd1/1(y) -> Sum2/1, Gain3/1
  Gain7/1 -> Sum3/2
  [El] -> 1+Sd1/2(El)
  Gain9/1 -> Integrator3/1
  Sum/1 -> Gain1/1
  Gain10/1 -> Sum5/3
  El/1 -> [El]
  Gain5/1 -> Sum2/3
  Sum2/1 -> Gain4/1
  id/1 -> Gain5/1
  [El] -> 1+Sd/2(El)
  Sum5/1 -> Gain9/1
  iq/1 -> Gain10/1
  ve/1 -> Sum/2
  Sum3/1 -> Gain6/1
  Gain8/1 -> Sum3/1
  [El] -> 1+Sq1/2(El)
  Integrator/1 -> 1+Sd/1(u)  "Eqs"
  Integrator2/1 -> 1+Sq2/1(u)  "Eds"
  Gain6/1 -> Integrator2/1
  Gain4/1 -> Integrator1/1
  [El] -> 1+Sq2/2(El)
  1+Sq1/1(y) -> Sum5/1, Gain8/1
  1+Sq2/1(y) -> Gain7/1, Sum5/2
  Sum1/1 -> ifd/1
  Integrator1/1 -> 1+Sd1/1(u), Eqss/1  "Eqs"
  Integrator3/1 -> Edss/1, 1+Sq1/1(u)  "Edss"

== system ANS_GFM_short_term/Synchronous Generator(GENTPJ)/Stator Equations ==
  Id : Inport
  Iq : Inport  Port=2
  Edss : Inport  Port=3
  Eqss : Inport  Port=4
  E_l : Inport  Port=5
  1+w : Inport  Port=6
  1+Sd : Subsystem
  1+Sq : Subsystem
  Constant : Constant  Value=Xl
  Gain1 : Gain  Gain=Ra
  Gain2 : Gain  Gain=Ra
  Gain3 : Gain  Gain=(Xdss-Xl)
  Gain4 : Gain  Gain=(Xqss-Xl)
  Product{,1..3} (4 alike) : Product
  Sum : Sum  Inputs=+-+
  Sum1 : Sum  Inputs=|++
  Sum2 : Sum  Inputs=++|
  Sum3 : Sum  Inputs=--+
  Vdterm : Outport
  Vqterm : Outport  Port=2
  wires:
  Id/1 -> Product2/1, Gain1/1, Gain3/1
  Product/1 -> Sum/1
  1+w/1 -> [omega]
  Product3/1 -> Sum1/1
  Gain1/1 -> Sum/2
  Sum1/1 -> Sum/3
  Sum3/1 -> Vqterm/1
  Sum/1 -> Vdterm/1
  Product1/1 -> Sum3/3
  Iq/1 -> Product3/2, Gain2/1, Gain4/1
  Gain2/1 -> Sum3/2
  Eqss/1 -> Product1/1
  Edss/1 -> Product/1
  1+Sd/1(y) -> Sum2/1
  Gain4/1 -> 1+Sq/1(u)
  Sum2/1 -> Sum3/1
  Constant/1 -> Product2/2, Product3/1
  Gain3/1 -> 1+Sd/1(u)
  Product2/1 -> Sum2/2
  [omega] -> Product/2
  [El] -> 1+Sd/2(El)
  [omega] -> Product1/2
  1+Sq/1(y) -> Sum1/2
  [El] -> 1+Sq/2(El)
  E_l/1 -> [El]

== system ANS_GFM_short_term/GFM Converter/Converter (modified by S. Liemann)/Subsystem1 ==
  Vabc : Inport
  Controlled Voltage Source2 : spsControlledVoltageSourceLib/Controlled Voltage Source  Initialize=on  Source_Type=AC  Amplitude=Umag_init  Phase=Uangle_init  Frequency=50  Measurements=None
  Controlled Voltage Source3 : spsControlledVoltageSourceLib/Controlled Voltage Source  Initialize=on  Source_Type=AC  Amplitude=Umag_init  Phase=Uangle_init-120  Frequency=50  Measurements=None
  Controlled Voltage Source4 : spsControlledVoltageSourceLib/Controlled Voltage Source  Initialize=on  Source_Type=AC  Amplitude=Umag_init  Phase=Uangle_init+120  Frequency=50  Measurements=None
  Demux : Demux  Outputs=3
  Ground : spsGroundLib/Ground  LConnTagsString=a
  a : PMIOPort  Side=Right
  b : PMIOPort  Port=2  Side=Right
  c : PMIOPort  Port=3  Side=Right
  wires:
  Demux/3 -> Controlled Voltage Source4/1
  Demux/2 -> Controlled Voltage Source3/1
  Demux/1 -> Controlled Voltage Source2/1
  Vabc/1 -> Demux/1
  connections:
  Controlled Voltage Source2/RConn1 -- a/RConn1
  Controlled Voltage Source4/LConn1 -- Controlled Voltage Source3/LConn1 -- Controlled Voltage Source2/LConn1 -- Ground/LConn1
  Controlled Voltage Source3/RConn1 -- b/RConn1
  Controlled Voltage Source4/RConn1 -- c/RConn1

== system ANS_GFM_short_term/GFM Converter/GFM controls/Droop Control ==
  w_b : Inport
  p_m : Inport  Port=2
  p_set : Inport  Port=3
  v_m : Inport  Port=4
  V_abc : Inport  Port=5
  anti-windup : Inport  Port=6
  dv_q : Inport  Port=7
  Enable : EnablePort
  Constant : Constant  Value=0
  Demux3 : Demux  Outputs=3
  Gain : Gain  Gain=kp_v_ac
  Gain1 : Gain  Gain=ki_v_ac
  Gain20 : Gain  Gain=m_p
  Integrator : Integrator  InitialCondition=V_d_int
  Integrator3 : Integrator  InitialCondition=angleV_LF
  LTI System1 : cstblocks/LTI System  sys=ss(A_pm,B_pm,C_pm,D_pm)  IC=[init_pm]
  Mux4 : Mux  Inputs=3
  Sqrt3 : Sqrt  SaturateOnIntegerOverflow=on
  Sum : Sum  Inputs=|++
  Sum1 : Sum  Inputs=-+|
  Sum3 : Sum  Inputs=+++  InputSameDT=on  SaturateOnIntegerOverflow=on  OutDataTypeStr=Inherit: Same as first input
  Sum7 : Sum  Inputs=|+-
  Sum8 : Sum  Inputs=+-+
  Switch2 : Switch  Criteria=u2 > Threshold
  abc to dq1 : spsabctodq0Lib/abc to dq0  Alignment=90 degrees behind phase A axis
  d²2 : Product  InputSameDT=on  RndMeth=Zero  SaturateOnIntegerOverflow=on  OutDataTypeStr=Inherit: Same as first input
  q0 : Constant  Value=0
  q²4 : Product  InputSameDT=on  RndMeth=Zero  SaturateOnIntegerOverflow=on  OutDataTypeStr=Inherit: Same as first input
  q²5 : Product  InputSameDT=on  RndMeth=Zero  SaturateOnIntegerOverflow=on  OutDataTypeStr=Inherit: Same as first input
  w_ref : Outport  VectorParamsAs1DForOutWhenUnconnected=off
  theta_ref : Outport  Port=2  VectorParamsAs1DForOutWhenUnconnected=off
  v_ref_dq0 : Outport  Port=3  VectorParamsAs1DForOutWhenUnconnected=off
  wires:
  LTI System1/1 -> Sum7/1
  Mux4/1 -> v_ref_dq0/1
  q0/1 -> Mux4/3, Mux4/2
  Sum8/1 -> Integrator3/1, w_ref/1
  Gain20/1 -> Sum8/2
  Sum7/1 -> Gain20/1
  p_set/1 -> Sum7/2
  w_b/1 -> Sum8/1
  V_abc/1 -> abc to dq1/1
  Integrator3/1 -> theta_ref/1, abc to dq1/2
  v_m/1 -> Sum1/2
  Sum/1 -> Mux4/1
  Sum1/1 -> Switch2/1, Gain/1
  Constant/1 -> Switch2/3
  Switch2/1 -> Gain1/1
  anti-windup/1 -> Switch2/2
  Gain/1 -> Sum/1
  Gain1/1 -> Integrator/1
  p_m/1 -> LTI System1/1
  Integrator/1 -> Sum/2
  abc to dq1/1 -> Demux3/1
  q²4/1 -> Sum3/2
  Demux3/3 -> q²5/2, q²5/1  "0"
  Demux3/2 -> q²4/2, q²4/1  "q"
  Demux3/1 -> d²2/2, d²2/1  "d"
  d²2/1 -> Sum3/1
  Sum3/1 -> Sqrt3/1
  q²5/1 -> Sum3/3
  Sqrt3/1 -> Sum1/1
  dv_q/1 -> Sum8/3

== system ANS_GFM_short_term/GFM Converter/GFM controls/Matching Control ==
  v_dc : Inport
  V_abc : Inport  Port=2
  v_m : Inport  Port=3
  anti-windup : Inport  Port=4
  dv_q : Inport  Port=5
  Enable : EnablePort
  Alpha-Beta-Zero to dq0 : spsAlphaBetaZerotodq0Lib/Alpha-Beta-Zero to dq0  Commented=on  Alignment=90 degrees behind phase A axis
      settings: SourceProductBaseCode=PS
  Constant : Constant  Value=0
  Constant1 : Constant  Value=0
  Constant2 : Constant  Commented=on  Value=0
  Demux2 : Demux  Outputs=3
  Fcn2 : Fcn  Commented=on  Expr=sin(u)
  Fcn3 : Fcn  Commented=on  Expr=-cos(u)
  Gain : Gain  Gain=kp_v_ac
  Gain1 : Gain  Gain=ki_v_ac
  Gain2 : Gain  Gain=1/Vdc_n
  Gain4 : Gain  Gain=w_b
  Integrator : Integrator  InitialCondition=V_d_int
  Integrator5 : Integrator  InitialCondition=angleV_LF
  Mux1 : Mux  Commented=on  Inputs=3
  Mux2 : Mux  Inputs=3
  Product3 : Product  Commented=on
  Product4 : Product  Commented=on
  Sqrt2 : Sqrt  SaturateOnIntegerOverflow=on
  Sum : Sum  Inputs=|++
  Sum1 : Sum  Inputs=-+|
  Sum2 : Sum  Inputs=+++  InputSameDT=on  SaturateOnIntegerOverflow=on  OutDataTypeStr=Inherit: Same as first input
  Sum3 : Sum  Inputs=|++
  Switch2 : Switch  Criteria=u2 > Threshold
  abc to dq1 : spsabctodq0Lib/abc to dq0  Alignment=90 degrees behind phase A axis
  d²2 : Product  InputSameDT=on  RndMeth=Zero  SaturateOnIntegerOverflow=on  OutDataTypeStr=Inherit: Same as first input
  q²4 : Product  InputSameDT=on  RndMeth=Zero  SaturateOnIntegerOverflow=on  OutDataTypeStr=Inherit: Same as first input
  q²5 : Product  InputSameDT=on  RndMeth=Zero  SaturateOnIntegerOverflow=on  OutDataTypeStr=Inherit: Same as first input
  w_ref : Outport  VectorParamsAs1DForOutWhenUnconnected=off
  theta_ref : Outport  Port=2  VectorParamsAs1DForOutWhenUnconnected=off
  v_ref_dq0 : Outport  Port=3  VectorParamsAs1DForOutWhenUnconnected=off
  wires:
  Sum/1 -> Mux2/1, Product4/1, Product3/2
  q²5/1 -> Sum2/3
  abc to dq1/1 -> Demux2/1
  Demux2/2 -> q²4/1, q²4/2  "q"
  d²2/1 -> Sum2/1
  q²4/1 -> Sum2/2
  Demux2/1 -> d²2/1, d²2/2  "d"
  Sum2/1 -> Sqrt2/1
  Demux2/3 -> q²5/1, q²5/2  "0"
  Sqrt2/1 -> Sum1/1
  V_abc/1 -> abc to dq1/1
  v_m/1 -> Sum1/2
  Mux1/1 -> Alpha-Beta-Zero to dq0/1
  Constant2/1 -> Mux1/3
  Product4/1 -> Mux1/2
  Product3/1 -> Mux1/1
  Fcn3/1 -> Product4/2
  Fcn2/1 -> Product3/1
  v_dc/1 -> Gain2/1
  Gain1/1 -> Integrator/1
  Gain/1 -> Sum/1
  Integrator/1 -> Sum/2
  anti-windup/1 -> Switch2/2
  Sum1/1 -> Gain/1, Switch2/1
  Constant/1 -> Switch2/3
  Gain2/1 -> Gain4/1
  Integrator5/1 -> abc to dq1/2, theta_ref/1, Alpha-Beta-Zero to dq0/2, Fcn3/1, Fcn2/1
  Switch2/1 -> Gain1/1
  Mux2/1 -> v_ref_dq0/1
  Constant1/1 -> Mux2/3, Mux2/2
  Gain4/1 -> Sum3/1
  Sum3/1 -> w_ref/1, Integrator5/1
  dv_q/1 -> Sum3/2

== system ANS_GFM_short_term/GFM Converter/GFM controls/VSM Control ==
  p_m : Inport
  p_set : Inport  Port=2
  v_m : Inport  Port=3
  V_abc : Inport  Port=4
  w_b : Inport  Port=5
  anti-windup : Inport  Port=6
  dv_q : Inport  Port=7
  Enable : EnablePort
  Constant : Constant  Value=0
  Demux3 : Demux  Outputs=3
  Gain : Gain  Gain=kp_v_ac
  Gain1 : Gain  Gain=ki_v_ac
  Gain17 : Gain  Gain=1/(w_b)
  Gain2 : Gain  Gain=1/(w_b)
  Gain5 : Gain  Gain=D_p
  Gain6 : Gain  Gain=1/J
  Gain8 : Gain  Gain=1/w_b
  Integrator : Integrator  InitialCondition=50*2*pi
  Integrator1 : Integrator  InitialCondition=V_d_int/(100*pi)^0
  Integrator2 : Integrator  InitialCondition=angleV_LF
  LTI System2 : cstblocks/LTI System  sys=ss(A_pm,B_pm,C_pm,D_pm)  IC=[init_pm]
  MATLAB Function1 : MATLAB Function  TreatAsAtomicUnit=on
  Sqrt3 : Sqrt  SaturateOnIntegerOverflow=on
  Sum : Sum  Inputs=+|+|-
  Sum1 : Sum  Inputs=-++
  Sum2 : Sum  Inputs=+|-
  Sum3 : Sum  Inputs=|++
  Sum4 : Sum  Inputs=+++  InputSameDT=on  SaturateOnIntegerOverflow=on  OutDataTypeStr=Inherit: Same as first input
  Sum5 : Sum  Inputs=|++
  Switch2 : Switch  Criteria=u2 > Threshold
  abc to dq1 : spsabctodq0Lib/abc to dq0  Alignment=90 degrees behind phase A axis
  abc to dq2 : spsabctodq0Lib/abc to dq0  Alignment=90 degrees behind phase A axis
  d²2 : Product  InputSameDT=on  RndMeth=Zero  SaturateOnIntegerOverflow=on  OutDataTypeStr=Inherit: Same as first input
  q²4 : Product  InputSameDT=on  RndMeth=Zero  SaturateOnIntegerOverflow=on  OutDataTypeStr=Inherit: Same as first input
  q²5 : Product  InputSameDT=on  RndMeth=Zero  SaturateOnIntegerOverflow=on  OutDataTypeStr=Inherit: Same as first input
  w_ref : Outport  VectorParamsAs1DForOutWhenUnconnected=off
  theta_ref : Outport  Port=2  VectorParamsAs1DForOutWhenUnconnected=off
  v_ref_dq0 : Outport  Port=3  VectorParamsAs1DForOutWhenUnconnected=off
  wires:
  v_m/1 -> Sum1/2
  V_abc/1 -> abc to dq1/1
  w_b/1 -> Sum2/1
  LTI System2/1 -> Gain17/1
  Integrator2/1 -> abc to dq1/2, MATLAB Function1/2(theta), abc to dq2/2, theta_ref/1
  Sum2/1 -> Gain5/1
  Sum/1 -> Gain6/1
  Gain2/1 -> Sum/2
  Gain17/1 -> Sum/3
  p_m/1 -> LTI System2/1
  p_set/1 -> Gain2/1
  Sum3/1 -> MATLAB Function1/1(M_fi_f)
  abc to dq2/1 -> v_ref_dq0/1
  Constant/1 -> Switch2/3
  Sum1/1 -> Switch2/1, Gain/1
  Integrator1/1 -> Sum3/2
  Gain/1 -> Sum3/1
  anti-windup/1 -> Switch2/2
  Gain1/1 -> Integrator1/1
  Switch2/1 -> Gain1/1
  Gain6/1 -> Integrator/1
  Gain5/1 -> Sum/1
  MATLAB Function1/1(e) -> abc to dq2/1
  Gain8/1 -> MATLAB Function1/3(w)
  abc to dq1/1 -> Demux3/1
  q²4/1 -> Sum4/2
  Demux3/3 -> q²5/2, q²5/1  "0"
  Demux3/2 -> q²4/2, q²4/1  "q"
  Demux3/1 -> d²2/2, d²2/1  "d"
  d²2/1 -> Sum4/1
  Sum4/1 -> Sqrt3/1
  q²5/1 -> Sum4/3
  Sqrt3/1 -> Sum1/1
  Sum5/1 -> Gain8/1, Sum2/2, w_ref/1, Integrator2/1
  dv_q/1 -> Sum5/2
  Integrator/1 -> Sum5/1

== system ANS_GFM_short_term/GFM Converter/GFM controls/dVOC  - kappa=pi//2 ==
  w_b : Inport
  p_m : Inport  Port=2
  p_set : Inport  Port=3
  v_m : Inport  Port=4
  q_m : Inport  Port=5
  q_set : Inport  Port=6
  anti-windup : Inport  Port=7
  dv_q : Inport  Port=8
  Enable : EnablePort
  APC : Subsystem
  Constant : Constant  Commented=on  Value=epsi
  Integrator1 : Integrator  InitialCondition=V_d_int
  Integrator3 : Integrator  InitialCondition=angleV_LF
  Multiply1 : Product
  Mux4 : Mux  Inputs=3
  P-AVR : Subsystem
  RPC : Subsystem
  Sum1 : Sum  Inputs=|++
  Sum4 : Sum  Inputs=|++
  Sum8 : Sum  Inputs=+++
  q0 : Constant  Value=0
  w_ref : Outport  VectorParamsAs1DForOutWhenUnconnected=off
  theta_ref : Outport  Port=2  VectorParamsAs1DForOutWhenUnconnected=off
  v_ref_dq0 : Outport  Port=3  VectorParamsAs1DForOutWhenUnconnected=off
  wires:
  Mux4/1 -> v_ref_dq0/1
  q0/1 -> Mux4/3, Mux4/2
  Sum8/1 -> Integrator3/1, w_ref/1
  w_b/1 -> Sum8/1
  Integrator3/1 -> theta_ref/1
  p_m/1 -> APC/1(p)
  p_set/1 -> APC/2(p*)
  APC/1(dw) -> Sum8/2
  q_m/1 -> RPC/1(q)
  q_set/1 -> RPC/2(q*)
  Integrator1/1 -> Sum1/1
  Sum4/1 -> Multiply1/1
  v_m/1 -> P-AVR/2(v*), RPC/4(v*), APC/4(v*)
  P-AVR/1(dv2) -> Sum4/2
  Constant/1 -> Sum1/2
  RPC/1(dv1) -> Sum4/1
  Sum1/1 -> Multiply1/2, APC/3(v), RPC/3(v), P-AVR/1(v), Mux4/1
  Multiply1/1 -> Integrator1/1
  dv_q/1 -> Sum8/3

== system ANS_GFM_short_term/GFM Converter/SECMs/SECM-1 ==
  Pset0 : Inport
  imax_flag : Inport  Port=2
  Vdq0 : Inport  Port=3
  Idq0_lim : Inport  Port=4
  Qset0 : Inport  Port=5
  Enable : EnablePort
  Demux{,1..3} (4 alike) : Demux  Outputs=2
  Demux4 : Demux  Outputs=3
  Gain : Gain  Gain=1/(1/(100*pi*C_f)/Zbase_new)
  Gain1 : Gain  Gain=1/V_m
  Product{1..5} (5 alike) : Product
  Selector{1..4} (4 alike) : Selector  InputPortWidth=3  IndexOptions=Index vector (dialog)  Indices=[1 2]  OutputSizes=1
  Sqrt3 : Sqrt  SaturateOnIntegerOverflow=on
  Sum : Sum  Inputs=|++
  Sum1 : Sum  Inputs=|++
  Sum2 : Sum  Inputs=|-+
  Sum3 : Sum  Inputs=+++  InputSameDT=on  SaturateOnIntegerOverflow=on  OutDataTypeStr=Inherit: Same as first input
  Switch1 : Switch  Criteria=u2 ~= 0
  Switch2 : Switch  Criteria=u2 ~= 0
  dq-Trafo : Gain  Gain=3/2/S_bc
  dq-Trafo1 : Gain  Gain=3/2/S_bc
  d²2 : Product  InputSameDT=on  RndMeth=Zero  SaturateOnIntegerOverflow=on  OutDataTypeStr=Inherit: Same as first input
  q²4 : Product  InputSameDT=on  RndMeth=Zero  SaturateOnIntegerOverflow=on  OutDataTypeStr=Inherit: Same as first input
  q²5 : Product  InputSameDT=on  RndMeth=Zero  SaturateOnIntegerOverflow=on  OutDataTypeStr=Inherit: Same as first input
  pset* : Outport
  qset* : Outport  Port=2
  wires:
  Product1/1 -> Sum1/1  "ohne vq"
  Selector1/1 -> Demux/1
  Demux/1 -> Product1/1
  Sum1/1 -> dq-Trafo/1  "alles"
  Demux1/1 -> Product1/2
  Demux/2 -> Product2/1
  Selector2/1 -> Demux1/1
  Product2/1 -> Sum1/2
  Demux1/2 -> Product2/2
  Idq0_lim/1 -> Selector4/1, Selector2/1
  imax_flag/1 -> Switch2/2, Switch1/2
  dq-Trafo/1 -> Switch2/3
  Pset0/1 -> Switch2/1
  Switch2/1 -> pset*/1
  Selector4/1 -> Demux3/1
  Sum2/1 -> dq-Trafo1/1
  Product4/1 -> Sum2/2
  Selector3/1 -> Demux2/1
  Product3/1 -> Sum2/1
  Demux2/1 -> Product3/1
  Demux3/2 -> Product3/2
  Demux3/1 -> Product4/1
  Demux2/2 -> Product4/2
  Qset0/1 -> Switch1/1
  Switch1/1 -> qset*/1
  Product5/1 -> Gain/1
  dq-Trafo1/1 -> Sum/1  "vd"
  Sum/1 -> Switch1/3
  q²5/1 -> Sum3/3
  q²4/1 -> Sum3/2
  Vdq0/1 -> Selector1/1, Selector3/1, Gain1/1
  Demux4/3 -> q²5/2, q²5/1  "0"
  Sum3/1 -> Sqrt3/1
  d²2/1 -> Sum3/1
  Demux4/1 -> d²2/2, d²2/1  "d"
  Demux4/2 -> q²4/2, q²4/1  "q"
  Sqrt3/1 -> Product5/2, Product5/1
  Gain1/1 -> Demux4/1
  Gain/1 -> Sum/2  "xcf"

== system ANS_GFM_short_term/GFM Converter/SECMs/SECM-2 ==
  note: N. Wiese, D. Duckwitz, M. Nuschke, Y. Zhang, and M. Braun, “Fault
      | operation of grid-forming converters with focus on system stability,”
      | 11th Solar & Storage Power System Integration Workshop (SIW 2021),
      | pp. 65–70, 2021.
  pset : Inport
  V_pu : Inport  Port=2
  Enable : EnablePort
  Product : Product
  Switch2 : Switch  Threshold=0.9
  pset* : Outport
  wires:
  pset/1 -> Product/1, Switch2/1
  Switch2/1 -> pset*/1
  V_pu/1 -> Switch2/2, Product/2
  Product/1 -> Switch2/3

== system ANS_GFM_short_term/GFM Converter/SECMs/SECM-3 ==
  note: L. Huang et al., “Transient stability analysis and control design of droopcontrolled
      | voltage source converters considering current limitation,”
      | IEEE Transactions on Smart Grid, vol. 10, no. 1, pp. 578–591, 2019.
  pset : Inport
  V_q_pu : Inport  Port=2
  Enable : EnablePort
  Gain : Gain  Gain=-Kpl
  pset* : Outport
  dv_q : Outport  Port=2
  wires:
  V_q_pu/1 -> Gain/1
  pset/1 -> pset*/1
  Gain/1 -> dv_q/1

== system ANS_GFM_short_term/GFM Converter/SECMs/SECM-4 ==
  note: A. Tayyebi, D. Groß, A. Anta, F. Kupzog, and F. D¨orfler, “Frequency
      | stability of synchronous machines and grid-forming power converters,”
      | IEEE Journal of Emerging and Selected Topics in Power Electronics,
      | vol. 8, no. 2, pp. 1004–1018, 2020.
  pset : Inport
  i_s_dq0 : Inport  Port=2
  Enable : EnablePort
  Constant3 : Constant  Value=idppu
  Dot Product : DotProduct  InputSameDT=on  OutDataTypeStr=Inherit: Inherit via internal rule
  Gain : Gain  Gain=[eye(2),zeros(2,1)]  Multiplication=Matrix(K*u) (u vector)
  Gain2 : Gain  Gain=1/(I_bc*sqrt(2))
  Gain4 : Gain  Gain=gamma
  Saturation : Saturate  UpperLimit=inf  LowerLimit=0
  Sqrt : Sqrt  SaturateOnIntegerOverflow=on
  Sum : Sum  Inputs=|+-
  Sum1 : Sum  Inputs=+-|
  pset* : Outport  VectorParamsAs1DForOutWhenUnconnected=off
  wires:
  Dot Product/1 -> Sqrt/1
  Gain/1 -> Dot Product/1, Dot Product/2
  Sqrt/1 -> Sum/1
  Sum/1 -> Saturation/1
  Saturation/1 -> Gain4/1
  Constant3/1 -> Sum/2
  Gain4/1 -> Sum1/2
  Sum1/1 -> pset*/1
  pset/1 -> Sum1/1
  i_s_dq0/1 -> Gain2/1
  Gain2/1 -> Gain/1
